simulink model "MARCH_demo"  (R2016a)
settings: Solver=FixedStepDiscrete  StartTime=0.0  StopTime=inf  FixedStep=0.001  RelTol=1e-3
InitFcn:
  | % Change dir to model location
  | cd(fileparts(which(bdroot)));
  | 
  | init_model
  | initialize_model_testingBlocks
StartFcn:
  | cd(fileparts(which(bdroot)));
StopFcn:
  | cd(fileparts(which(bdroot)));
model workspace (MAT data in the model file):
  localValue = 1
  targetValue = 0
undefined symbols (not defined in the file or in its folder): Hip_HAA, Left_Leg, Right_Leg
libraries: xpcethercatlib x54, slrtlib x7, aerolibanimutils x1, dspnetwork x1
CloseFcn:
  | cd(fileparts(which(bdroot)));
settings Model: Creator=march  LastModifiedBy=Nathan
settings SolverCC: EnableConcurrentExecution=on
settings DataIOCC: SaveFormat=StructureWithTime
settings OptimizationCC: BlockReduction=off  OptimizeBlockIOStorage=off  BufferReuse=off  GlobalBufferReuse=off  ExpressionFolding=off  LocalBlockOutputs=off
settings HardwareCC: ProdBitPerPointer=32  ProdLargestAtomicFloat=None  ProdWordSize=32  ProdLongLongMode=on  ProdHWDeviceType=Generic->32-bit x86 compatible
settings RTWCC: SystemTargetFile=slrt.tlc  TemplateMakefile=slrt_default_tmf  Description=Simulink Real-Time
settings SimulinkRealTimeCC: xPCisDownloadable=off  xPCisModelTimeout=off  xPCModelTimeoutSecs=30

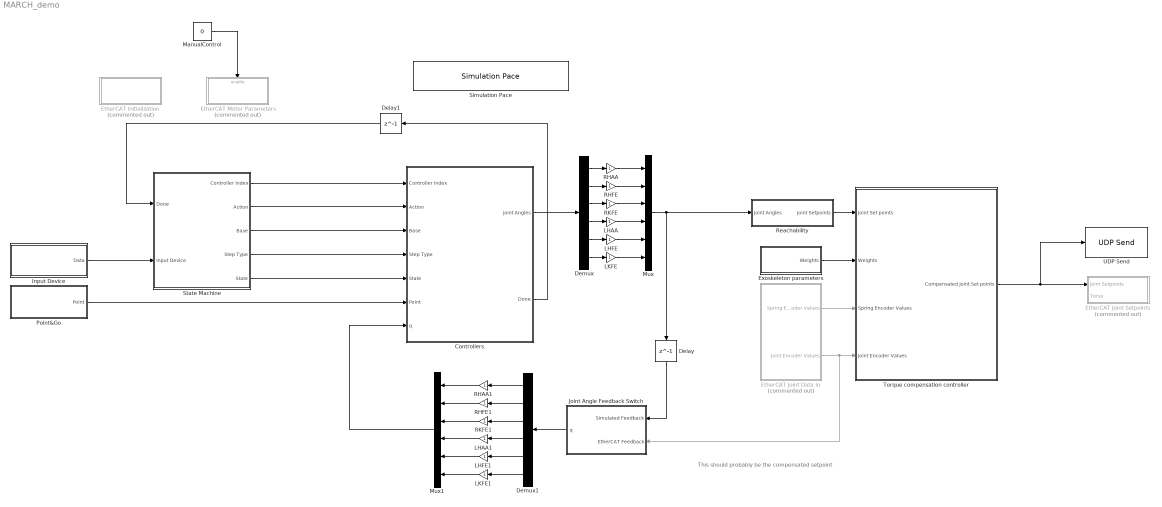
== system MARCH_demo ==
  note: This should probably be the compensated setpoint
  Controllers : Subsystem
  Delay : Delay  DelayLength=1
  Delay1 : Delay  DelayLength=1
  Demux : Demux  Outputs=6
  Demux1 : Demux  Outputs=6
  EtherCAT Initialization : Subsystem  Commented=on
  EtherCAT Joint Data In : Subsystem  Commented=on
  EtherCAT Joint Setpoints : Subsystem  Commented=on
  EtherCAT Motor Parameters : Subsystem  Commented=on
  Exoskeleton parameters : Subsystem
  Input Device : Subsystem
  Joint Angle Feedback Switch : Subsystem
  LHAA : Gain
  LHAA1 : Gain
  LHFE : Gain
  LHFE1 : Gain
  LKFE : Gain
  LKFE1 : Gain
  ManualControl : Constant  Value=0
  Mux : Mux  Inputs=6
  Mux1 : Mux  Inputs=6
  Point&Go : Subsystem
  RHAA : Gain
  RHAA1 : Gain
  RHFE : Gain
  RHFE1 : Gain
  RKFE : Gain
  RKFE1 : Gain
  Reachability : Subsystem
  Simulation Pace : aerolibanimutils/Simulation Pace  SimulationPace=1  SleepMode=MATLAB Thread  OutputPaceError=off  SampleTime=-1
  State Machine : Subsystem
  Torque compensation controller : Subsystem
  UDP Send : dspnetwork/UDP Send  remoteURL='127.0.0.1'  remotePort=25000  localURL='0.0.0.0'  localPortSource=Automatically determine  localPort=-1  sampletime=-1  separateLengthPort=0
  wires:
  Torque compensation controller/1(Compensated Joint Set points) -> UDP Send/1, EtherCAT Joint Setpoints/1(Joint Setpoints)
  Reachability/1(Joint Setpoints) -> Torque compensation controller/1(Joint Set points)
  EtherCAT Joint Data In/1(Spring Encoder Values) -> Torque compensation controller/3(Spring Encoder Values)
  EtherCAT Joint Data In/2(Joint Encoder Values) -> Joint Angle Feedback Switch/2(EtherCAT Feedback), Torque compensation controller/4(Joint Encoder Values)
  Exoskeleton parameters/1(Weights) -> Torque compensation controller/2(Weights)
  Delay/1 -> Joint Angle Feedback Switch/1(Simulated Feedback)
  Point&Go/1(Point) -> Controllers/6(Point)
  Input Device/1(Data) -> State Machine/2(Input Device)
  Controllers/2(Done) -> Delay1/1
  State Machine/4(Step Type) -> Controllers/4(Step Type)
  State Machine/2(Action) -> Controllers/2(Action)
  State Machine/3(Base) -> Controllers/3(Base)
  State Machine/1(Controller Index) -> Controllers/1(Controller Index)
  State Machine/5(State) -> Controllers/5(State)
  Delay1/1 -> State Machine/1(Done)
  Demux/1 -> RHAA/1
  Demux/2 -> RHFE/1
  Demux/3 -> RKFE/1
  Demux/4 -> LHAA/1
  Demux/5 -> LHFE/1
  Demux/6 -> LKFE/1
  Controllers/1(joint Angles) -> Demux/1
  Mux/1 -> Reachability/1(Joint Angles), Delay/1
  RHAA/1 -> Mux/1
  RHFE/1 -> Mux/2
  RKFE/1 -> Mux/3
  LHAA/1 -> Mux/4
  LHFE/1 -> Mux/5
  LKFE/1 -> Mux/6
  Demux1/1 -> RHAA1/1
  Demux1/2 -> RHFE1/1
  Demux1/3 -> RKFE1/1
  Demux1/4 -> LHAA1/1
  Demux1/5 -> LHFE1/1
  Demux1/6 -> LKFE1/1
  RHFE1/1 -> Mux1/2
  RKFE1/1 -> Mux1/3
  LHAA1/1 -> Mux1/4
  LHFE1/1 -> Mux1/5
  LKFE1/1 -> Mux1/6
  RHAA1/1 -> Mux1/1
  Joint Angle Feedback Switch/1(q) -> Demux1/1
  Mux1/1 -> Controllers/7(q)
  ManualControl/1 -> EtherCAT Motor Parameters/Enable

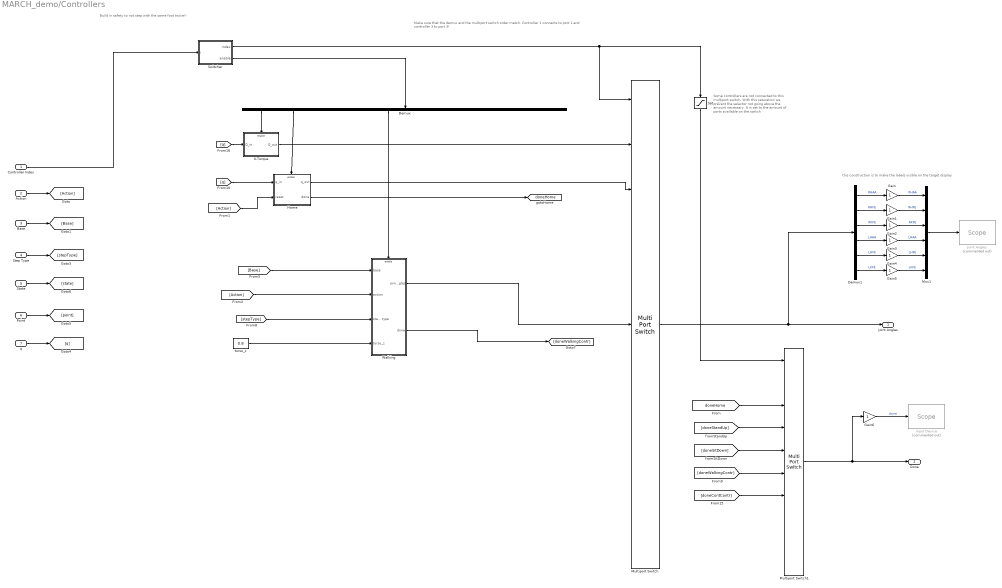
== system MARCH_demo/Controllers ==
  note: Some controllers are not connected to this multiport switch. With this saturation we prevent the selector not going above the amount necessary. It is set to the amount of ports available on the switch
  note: Build in safety to not step with the same
      | foot twice!!
  note: Make sure that the demux and the multiport switch order match.
      | Controller 1 connects to port 1 and controller 3 to port 3!
  note: this construction is to make the labels visible on the target display
  Controller Index : Inport
  Action : Inport  Port=2
  Base : Inport  Port=3
  Step Type : Inport  Port=4
  State : Inport  Port=5
  Point : Inport  Port=6
  q : Inport  Port=7
  0-Torque : Subsystem
  Demux : Demux  Outputs=10
  Demux1 : Demux  Outputs=6
  Gain{,1..6} (7 alike) : Gain
  Home : Subsystem
  Input Device : slrtlib/Displays and Logging/Scope   Commented=on  scopeno=4  scopetype=Target  autostart=on  viewmode=Graphical sliding  formatstr='%15.6f'  grid=on  ylimits=[0,0]  nosamples=25000  noprepostsamples=0  interleave=1  triggermode=FreeRun  triggersignal=1  trigsignalfromport=off  triggerlevel=0.0  triggerslope=Either  triggerscope=1  triggersample=0  filename=data.dat  mode=Lazy  writesize=512  autorestart=off  dynamicfilemode=off  maxwritefilesize=512*1024^2
  Joint Angles : slrtlib/Displays and Logging/Scope   Commented=on  scopeno=3  scopetype=Target  autostart=on  viewmode=Graphical sliding  formatstr='%15.6f'  grid=on  ylimits=[0,0]  nosamples=25000  noprepostsamples=0  interleave=1  triggermode=FreeRun  triggersignal=1  trigsignalfromport=off  triggerlevel=0.0  triggerslope=Either  triggerscope=1  triggersample=0  filename=data.dat  mode=Lazy  writesize=512  autorestart=off  dynamicfilemode=off  maxwritefilesize=512*1024^2
  Multiport Switch : MultiPortSwitch  Inputs=10
  Multiport Switch1 : MultiPortSwitch  Inputs=8  DataPortForDefault=Additional data port
  Mux1 : Mux  Inputs=6
  Saturation : Saturate  UpperLimit=8  LowerLimit=1
  Switcher : MATLAB Function  TreatAsAtomicUnit=on
  Walking : Subsystem
  torso_z : Constant  Value=0.8
  joint Angles : Outport
  Done : Outport  Port=2
  tag scope: doneHome=global
  wires:
  Switcher/1(index) -> Saturation/1, Multiport Switch/1
  Switcher/2(enable) -> Demux/1
  Multiport Switch1/1 -> Gain6/1, Done/1
  Saturation/1 -> Multiport Switch1/1
  Demux/1 -> 0-Torque/Enable
  Demux/5 -> Walking/Enable
  0-Torque/1(Q_out) -> Multiport Switch/2
  Home/1(q_out) -> Multiport Switch/3
  Walking/1(joint Angles) -> Multiport Switch/6
  Action/1 -> [Action]
  Base/1 -> [Base]
  Point/1 -> [point]
  q/1 -> [q]
  Step Type/1 -> [stepType]
  [Action] -> Walking/2(action)
  [Base] -> Walking/1(base)
  [stepType] -> Walking/3(step type)
  Walking/2(done) -> [doneWalkingContr]
  [doneWalkingContr] -> Multiport Switch1/6
  [doneContContr] -> Multiport Switch1/7
  State/1 -> [state]
  Home/2(done) -> [doneHome]
  [doneStandUp] -> Multiport Switch1/4
  Multiport Switch/1 -> joint Angles/1, Demux1/1
  Demux1/1 -> Gain/1  "RHAA"
  Demux1/2 -> Gain1/1  "RHFE"
  Demux1/3 -> Gain2/1  "RKFE"
  Demux1/4 -> Gain3/1  "LHAA"
  Demux1/5 -> Gain4/1  "LHFE"
  Demux1/6 -> Gain5/1  "LKFE"
  Mux1/1 -> Joint Angles/1
  Gain/1 -> Mux1/1  "RHAA"
  Gain1/1 -> Mux1/2  "RHFE"
  Gain2/1 -> Mux1/3  "RKFE"
  Gain3/1 -> Mux1/4  "LHAA"
  Gain4/1 -> Mux1/5  "LHFE"
  Gain5/1 -> Mux1/6  "LKFE"
  Gain6/1 -> Input Device/1  "done"
  [doneSitDown] -> Multiport Switch1/5
  Controller Index/1 -> Switcher/1(i)
  torso_z/1 -> Walking/4(torso_z)
  [q] -> 0-Torque/1(Q_in)
  [doneHome] -> Multiport Switch1/3
  [Action] -> Home/2(reset)
  [q] -> Home/1(q_in)
  Demux/2 -> Home/Enable

== system MARCH_demo/EtherCAT Initialization ==
  EtherCAT Init : xpcethercatlib/EtherCAT Init   Priority=0  config_file=C:\Users\march\Documents\Software\MATLAB\simulink-models\EtherCAT Config Files\full_setup_v1.0.xml  device_id=0  pci_bus=2  pci_slot=0  dctuning=0  enaDebug=off  enaDC=on  errLink=on  masterDbg=on  stateChgDbg=on  baseClock=off  masterCfg=off  logFile='c:\dbglog.txt'  sample_time=0.001000
  EtherCAT Init1 : xpcethercatlib/EtherCAT Init   Priority=0  config_file=C:\Users\march\Documents\Software\MATLAB\simulink-models\EtherCAT Config files\input_device.xml  device_id=1  pci_bus=3  pci_slot=0  dctuning=1  enaDebug=off  enaDC=on  errLink=on  masterDbg=on  stateChgDbg=on  baseClock=off  masterCfg=off  logFile='c:\dbglog.txt'  sample_time=0.001000
  Terminator : Terminator
  Terminator1 : Terminator
  wires:
  EtherCAT Init/1 -> Terminator/1
  EtherCAT Init1/1 -> Terminator1/1

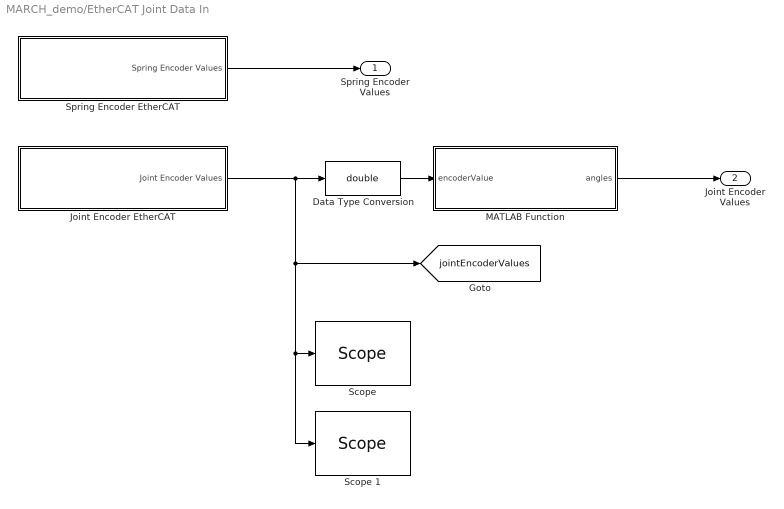
== system MARCH_demo/EtherCAT Joint Data In ==
  Data Type Conversion : DataTypeConversion  OutDataTypeStr=double
  Joint Encoder EtherCAT : Subsystem
  MATLAB Function : MATLAB Function  TreatAsAtomicUnit=on
  "Scope " : slrtlib/Displays and Logging/Scope   scopeno=6  scopetype=Target  autostart=on  viewmode=Graphical sliding  formatstr='%15.6f'  grid=on  ylimits=[0,0]  nosamples=25000  noprepostsamples=0  interleave=1  triggermode=FreeRun  triggersignal=1  trigsignalfromport=off  triggerlevel=0.0  triggerslope=Either  triggerscope=1  triggersample=0  filename=data.dat  mode=Lazy  writesize=512  autorestart=off  dynamicfilemode=off  maxwritefilesize=512*1024^2
  Scope 1 : slrtlib/Displays and Logging/Scope   scopeno=7  scopetype=Target  autostart=on  viewmode=Numerical  formatstr='%15.6f'  grid=on  ylimits=[0,0]  nosamples=3  noprepostsamples=0  interleave=1  triggermode=FreeRun  triggersignal=1  trigsignalfromport=off  triggerlevel=0.0  triggerslope=Either  triggerscope=1  triggersample=0  filename=data.dat  mode=Lazy  writesize=512  autorestart=off  dynamicfilemode=off  maxwritefilesize=512*1024^2
  Spring Encoder EtherCAT : Subsystem
  Spring Encoder Values : Outport
  Joint Encoder Values : Outport  Port=2
  tag scope: jointEncoderValues=global
  wires:
  Spring Encoder EtherCAT/1(Spring Encoder Values) -> Spring Encoder Values/1
  Joint Encoder EtherCAT/1(Joint Encoder Values) -> Data Type Conversion/1, Scope 1/1, "Scope "/1, [jointEncoderValues]
  MATLAB Function/1(angles) -> Joint Encoder Values/1
  Data Type Conversion/1 -> MATLAB Function/1(encoderValue)

== system MARCH_demo/EtherCAT Joint Setpoints ==
  Joint Setpoints : Inport
  Torso : Inport  Port=2
  Subsystem : Subsystem
  exoskeleton : Subsystem
  wires:
  Joint Setpoints/1 -> Subsystem/1(Joint Setpoints), exoskeleton/1(Joint setpoints)
  Torso/1 -> Subsystem/2(Torso)

== system MARCH_demo/EtherCAT Motor Parameters ==
  Enable : EnablePort
  Hips : Subsystem
  Left Leg : Subsystem
  Right Leg : Subsystem

== system MARCH_demo/Exoskeleton parameters ==
  Constant : Constant
  Weights : Outport
  wires:
  Constant/1 -> Weights/1

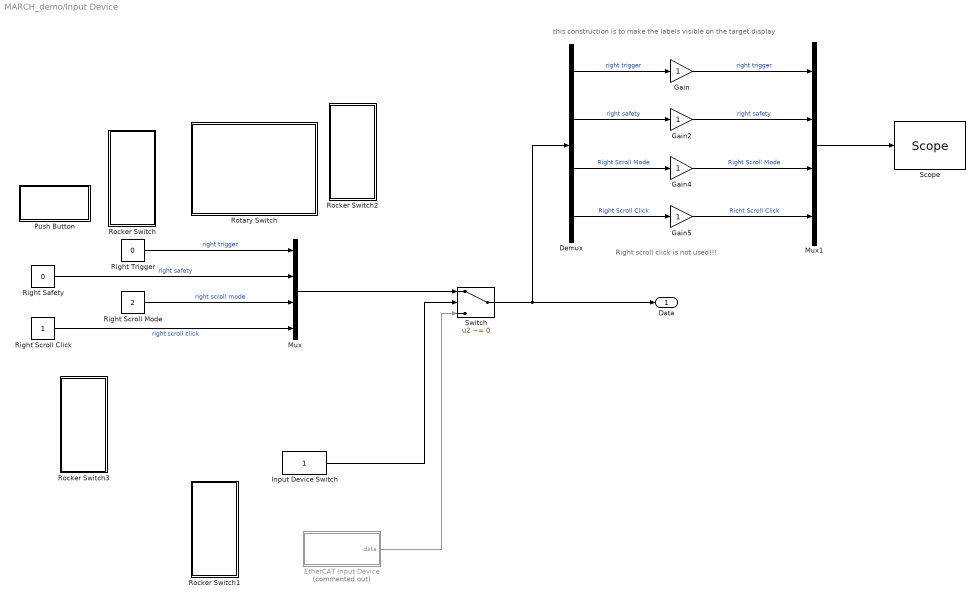
== system MARCH_demo/Input Device ==
  note: Right scroll click is not used!!!
  note: this construction is to make the labels visible on the target display
  Demux : Demux
  EtherCAT Input Device : Subsystem  Commented=on
  Gain{,2,4..5} (4 alike) : Gain
  Input Device Switch : Constant
  Mux : Mux
  Mux1 : Mux
  Push Button : Subsystem  DialogController=hmiCreateDDGDialog  IsWebBlock=on  mask(MWDashboardBlock){webBlockId=b5386708-d25b-47fc-ba10-cbba45de8cf4, webBlockType=pushbutton, ShowInLibBrwoser=on, ShowInitialText=on, HMISrcModelName=MARCH_demo}
      mask prompts: webBlockId "WebBlock Id"; webBlockType "WebBlock Type"; HMISrcModelName "Source Model"
      mask Help: helpview([docroot '/mapfiles/simulink.map'], 'hmi_push_button')
      mask Display:
      | model = bdroot(gcb);
      | if strcmp(get_param(model,'BlockDiagramType'), 'library')
      |     image([(matlabroot) '/toolbox/simulink/hmi/icons/PushButton.png']);
      | end
  Right Safety : Constant  Value=0
  Right Scroll Click : Constant
  Right Scroll Mode : Constant  Value=2
  Right Trigger : Constant  Value=0
  Rocker Switch : Subsystem  DialogController=hmiCreateDDGDialog  IsWebBlock=on  mask(MWDashboardBlock){webBlockId=45a61409-3ea3-4c23-95e6-fecf4e0aa3e0, webBlockType=rockerswitch, ShowInLibBrowser=on, ShowInitialText=on, HMISrcModelName=MARCH_demo}
      mask prompts: webBlockId "WebBlock Id"; webBlockType "WebBlock Type"; HMISrcModelName "Source Model"
      mask Help: helpview([docroot '/mapfiles/simulink.map'], 'hmi_rocker_switch')
      mask Display:
      | if strcmp(get_param(bdroot(gcb),'BlockDiagramType'), 'library')
      |     image([(matlabroot) '/toolbox/simulink/hmi/icons/RockerSwitch.png']);
      | end
  Rocker Switch1 : Subsystem  DialogController=hmiCreateDDGDialog  IsWebBlock=on  mask(MWDashboardBlock){webBlockId=cefc90cf-8074-4f09-bdc6-770b32cfa93a, webBlockType=rockerswitch, ShowInLibBrowser=on, ShowInitialText=on, HMISrcModelName=MARCH_demo}
      mask prompts: webBlockId "WebBlock Id"; webBlockType "WebBlock Type"; HMISrcModelName "Source Model"
      mask Help: helpview([docroot '/mapfiles/simulink.map'], 'hmi_rocker_switch')
      mask Display:
      | if strcmp(get_param(bdroot(gcb),'BlockDiagramType'), 'library')
      |     image([(matlabroot) '/toolbox/simulink/hmi/icons/RockerSwitch.png']);
      | end
  Rocker Switch2 : Subsystem  DialogController=hmiCreateDDGDialog  IsWebBlock=on  mask(MWDashboardBlock){webBlockId=9c410da0-0f2d-4180-a6e0-51db4255d255, webBlockType=rockerswitch, ShowInLibBrowser=on, ShowInitialText=on, HMISrcModelName=MARCH_demo}
      mask prompts: webBlockId "WebBlock Id"; webBlockType "WebBlock Type"; HMISrcModelName "Source Model"
      mask Help: helpview([docroot '/mapfiles/simulink.map'], 'hmi_rocker_switch')
      mask Display:
      | if strcmp(get_param(bdroot(gcb),'BlockDiagramType'), 'library')
      |     image([(matlabroot) '/toolbox/simulink/hmi/icons/RockerSwitch.png']);
      | end
  Rocker Switch3 : Subsystem  DialogController=hmiCreateDDGDialog  IsWebBlock=on  mask(MWDashboardBlock){webBlockId=f322042e-cbf0-407d-b585-24a2480925c8, webBlockType=rockerswitch, ShowInLibBrowser=on, ShowInitialText=on, HMISrcModelName=MARCH_demo}
      mask prompts: webBlockId "WebBlock Id"; webBlockType "WebBlock Type"; HMISrcModelName "Source Model"
      mask Help: helpview([docroot '/mapfiles/simulink.map'], 'hmi_rocker_switch')
      mask Display:
      | if strcmp(get_param(bdroot(gcb),'BlockDiagramType'), 'library')
      |     image([(matlabroot) '/toolbox/simulink/hmi/icons/RockerSwitch.png']);
      | end
  Rotary Switch : Subsystem  DialogController=hmiCreateDDGDialog  IsWebBlock=on  mask(MWDashboardBlock){webBlockId=2d14d417-f18b-4bf4-9f2c-b9e5fd3a8913, webBlockType=discreteknob, ShowInLibBrowser=on, ShowInitialText=on, HMISrcModelName=MARCH_demo}
      mask prompts: webBlockId "WebBlock Id"; webBlockType "WebBlock Type"; HMISrcModelName "Source Model"
      mask Help: helpview([docroot '/mapfiles/simulink.map'], 'hmi_rotary_switch')
      mask Display:
      | model = bdroot(gcb);
      | if strcmp(get_param(model,'BlockDiagramType'), 'library')
      |     image([(matlabroot) '/toolbox/simulink/hmi/icons/DiscreteKnob.png']);
      | end
  "Scope " : slrtlib/Displays and Logging/Scope   scopeno=1  scopetype=Target  autostart=on  viewmode=Numerical  formatstr='%15.6f'  grid=on  ylimits=[0,0]  nosamples=3  noprepostsamples=0  interleave=1  triggermode=FreeRun  triggersignal=1  trigsignalfromport=off  triggerlevel=0.0  triggerslope=Either  triggerscope=1  triggersample=0  filename=data.dat  mode=Lazy  writesize=512  autorestart=off  dynamicfilemode=off  maxwritefilesize=512*1024^2
  Switch : Switch  Criteria=u2 ~= 0
  Data : Outport
  wires:
  Input Device Switch/1 -> Switch/2
  EtherCAT Input Device/1(data) -> Switch/3
  Right Scroll Mode/1 -> Mux/3  "right scroll mode"
  Right Scroll Click/1 -> Mux/4  "right scroll click"
  Right Trigger/1 -> Mux/1  "right trigger"
  Right Safety/1 -> Mux/2  "right safety"
  Demux/1 -> Gain/1  "right trigger"
  Demux/2 -> Gain2/1  "right safety"
  Demux/3 -> Gain4/1  "Right Scroll Mode"
  Demux/4 -> Gain5/1  "Right Scroll Click"
  Gain/1 -> Mux1/1  "right trigger"
  Gain2/1 -> Mux1/2  "right safety"
  Gain4/1 -> Mux1/3  "Right Scroll Mode"
  Gain5/1 -> Mux1/4  "Richt Scroll Click"
  Switch/1 -> Data/1, Demux/1
  Mux/1 -> Switch/1
  Mux1/1 -> "Scope "/1

== system MARCH_demo/Joint Angle Feedback Switch ==
  Simulated Feedback : Inport
  EtherCAT Feedback : Inport  Port=2
  Local : Constant  Value=localValue
  Switch : Switch  Criteria=u2 ~= 0
  q : Outport
  wires:
  EtherCAT Feedback/1 -> Switch/3
  Switch/1 -> q/1
  Simulated Feedback/1 -> Switch/1
  Local/1 -> Switch/2

== system MARCH_demo/Point&Go ==
  note: For now, always use dummy point and go data even during target runs
  EtherCAT Point&Go : Subsystem  Commented=on
  Local : Constant  Value=localValue
  Point & Go Point : Constant  Value=[0.1 -0.3 0]
  Switch : Switch  Criteria=u2 ~= 0
  Point : Outport
  wires:
  EtherCAT Point&Go/1(Point&Go Data) -> Switch/3
  Local/1 -> Switch/2
  Switch/1 -> Point/1
  Point & Go Point/1 -> Switch/1

== system MARCH_demo/Reachability ==
  Joint Angles : Inport
  Data Type Conversion : DataTypeConversion  OutDataTypeStr=uint32
  MATLAB Function : MATLAB Function  Commented=on  TreatAsAtomicUnit=on
  Terminator2 : Terminator  Commented=on
  Joint Setpoints : Outport
  tag scope: jointSetpoints=global
  wires:
  MATLAB Function/2(err) -> Terminator2/1
  Data Type Conversion/1 -> [jointSetpoints]
  Joint Angles/1 -> Data Type Conversion/1, Joint Setpoints/1

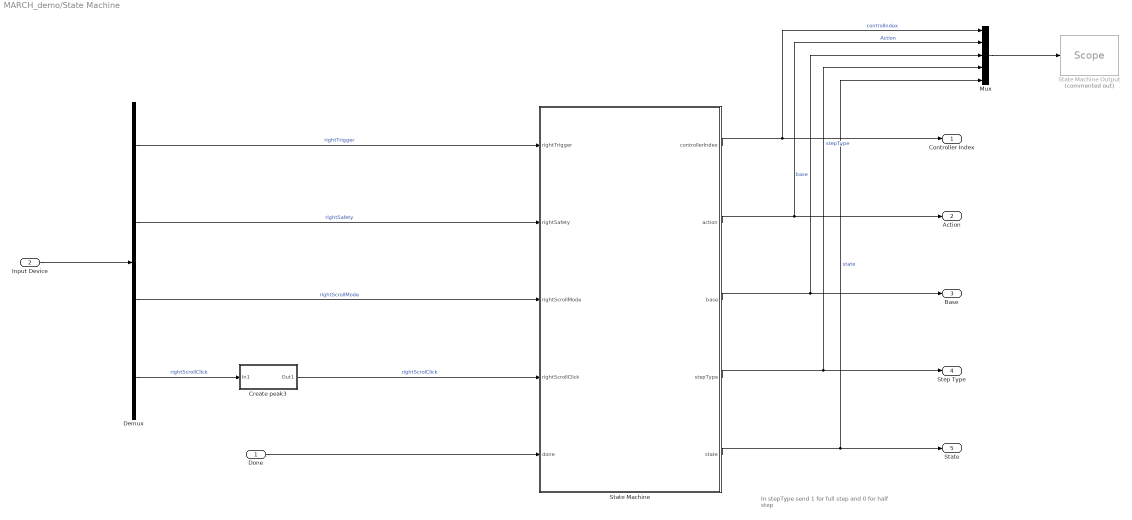
== system MARCH_demo/State Machine ==
  note: In stepType send 1 for full step and 0 for half step
  Done : Inport
  Input Device : Inport  Port=2
  Create peak3 : Subsystem
  Demux : Demux
  Mux : Mux  Inputs=5
  State Machine : Stateflow chart  TreatAsAtomicUnit=on
  State Machine Output : slrtlib/Displays and Logging/Scope   Commented=on  scopeno=2  scopetype=Target  autostart=on  viewmode=Numerical  formatstr='%15.6f'  grid=on  ylimits=[0,0]  nosamples=25  noprepostsamples=0  interleave=1  triggermode=FreeRun  triggersignal=1  trigsignalfromport=off  triggerlevel=0.0  triggerslope=Either  triggerscope=1  triggersample=0  filename=data.dat  mode=Lazy  writesize=512  autorestart=off  dynamicfilemode=off  maxwritefilesize=512*1024^2
  Controller Index : Outport
  Action : Outport  Port=2
  Base : Outport  Port=3
  Step Type : Outport  Port=4
  State : Outport  Port=5
  wires:
  Demux/2 -> State Machine/2(rightSafety)  "rightSafety"
  Demux/4 -> Create peak3/1(In1)  "rightScrollClick"
  Demux/1 -> State Machine/1(rightTrigger)  "rightTrigger"
  Create peak3/1(Out1) -> State Machine/4(rightScrollClick)  "rightScrolClick"
  Input Device/1 -> Demux/1
  Done/1 -> State Machine/5(done)
  State Machine/5(state) -> Mux/5, State/1  "state"
  State Machine/1(controllerIndex) -> Mux/1, Controller Index/1  "controlIndex"
  State Machine/2(action) -> Mux/2, Action/1  "Action"
  State Machine/3(base) -> Mux/3, Base/1  "base"
  State Machine/4(stepType) -> Mux/4, Step Type/1  "stepType"
  Mux/1 -> State Machine Output/1
  Demux/3 -> State Machine/3(rightScrollMode)  "rightScrollMode"

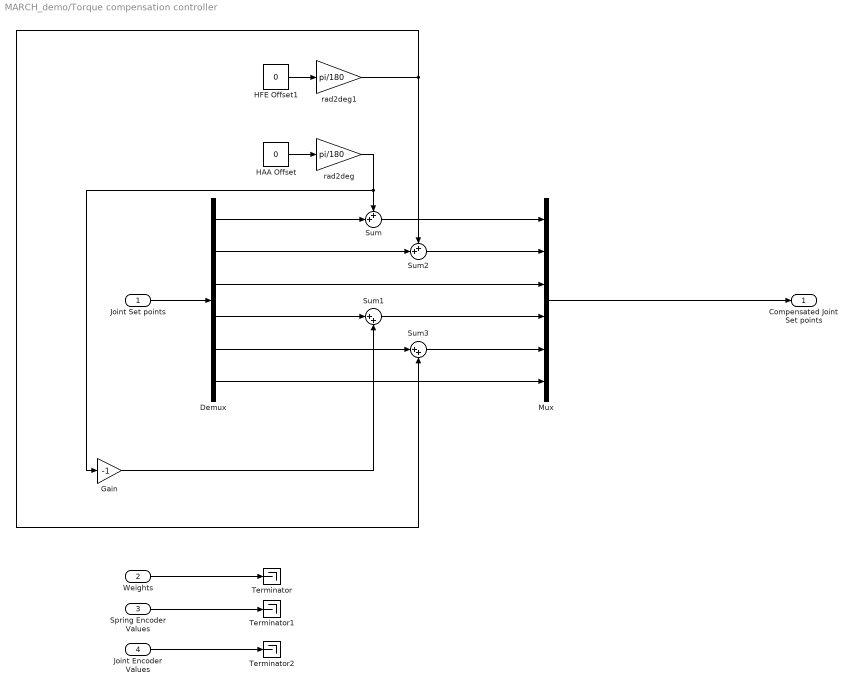
== system MARCH_demo/Torque compensation controller ==
  Joint Set points : Inport
  Weights : Inport  Port=2
  Spring Encoder Values : Inport  Port=3
  Joint Encoder Values : Inport  Port=4
  Demux : Demux  Outputs=6
  Gain : Gain  Gain=-1
  HAA Offset : Constant  Value=0
  HFE Offset1 : Constant  Value=0
  Mux : Mux  Inputs=6
  Sum : Sum  Inputs=++|
  Sum1 : Sum  Inputs=|++
  Sum2 : Sum  Inputs=++|
  Sum3 : Sum  Inputs=|++
  Terminator : Terminator
  Terminator1 : Terminator
  Terminator2 : Terminator
  rad2deg : Gain  Gain=pi/180
  rad2deg1 : Gain  Gain=pi/180
  Compensated Joint Set points : Outport
  wires:
  Joint Encoder Values/1 -> Terminator2/1
  Spring Encoder Values/1 -> Terminator1/1
  Weights/1 -> Terminator/1
  Joint Set points/1 -> Demux/1
  Demux/1 -> Sum/2
  Mux/1 -> Compensated Joint Set points/1
  Sum/1 -> Mux/1
  rad2deg/1 -> Gain/1, Sum/1
  HAA Offset/1 -> rad2deg/1
  Demux/2 -> Sum2/2
  Demux/3 -> Mux/3
  Sum1/1 -> Mux/4
  Demux/5 -> Sum3/1
  Demux/6 -> Mux/6
  Demux/4 -> Sum1/1
  Gain/1 -> Sum1/2
  HFE Offset1/1 -> rad2deg1/1
  Sum2/1 -> Mux/2
  Sum3/1 -> Mux/5
  rad2deg1/1 -> Sum2/1, Sum3/2

== system MARCH_demo/Controllers/0-Torque ==
  note: Since we don't control joint angles but motor velocity we just send dummy joint angles instead. This is a 1x6 vector of zeros.
  Q_in : Inport
  Enable : EnablePort  StatesWhenEnabling=reset
  Constant1 : Constant  Value=[0 0 0 0 0 0 ]  OutDataTypeStr=uint8
  Motor enable : Subsystem  Commented=on
  Q_out : Outport  InitialOutput=[0 0 0 0 0 0]
  wires:
  Q_in/1 -> Q_out/1
  Constant1/1 -> Motor enable/1(MotorEnableFlag)

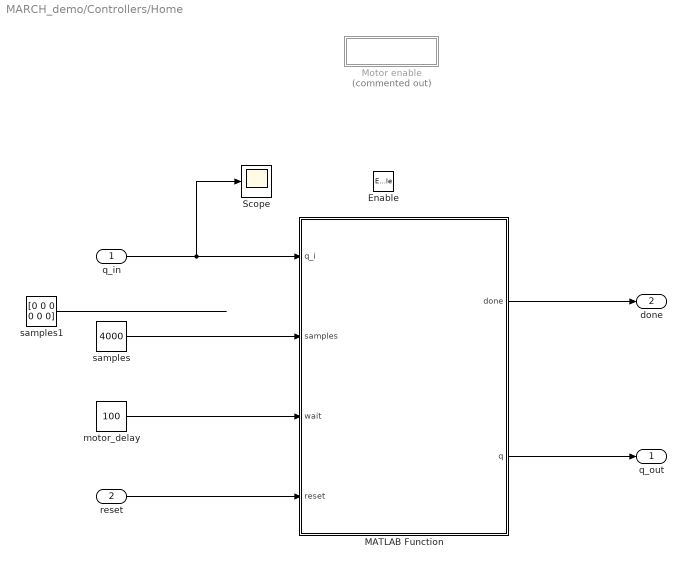
== system MARCH_demo/Controllers/Home ==
  q_in : Inport
  reset : Inport  Port=2
  Enable : EnablePort
  MATLAB Function : MATLAB Function  TreatAsAtomicUnit=on
  Motor enable : Subsystem  Commented=on
  Scope : Scope
  motor_delay : Constant  Value=100
  samples : Constant  Value=4000
  samples1 : Constant  Value=[0 0 0 0 0 0]
  q_out : Outport
  done : Outport  Port=2
  wires:
  MATLAB Function/1(done) -> done/1
  samples/1 -> MATLAB Function/2(samples)
  samples1/1 -> ?
  motor_delay/1 -> MATLAB Function/3(wait)
  MATLAB Function/2(q) -> q_out/1
  q_in/1 -> Scope/1, MATLAB Function/1(q_i)
  reset/1 -> MATLAB Function/4(reset)

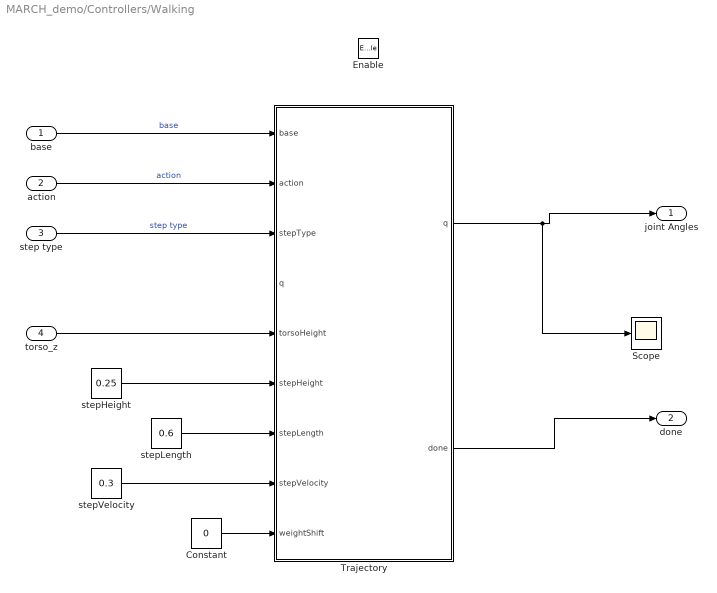
== system MARCH_demo/Controllers/Walking ==
  base : Inport
  action : Inport  Port=2
  step type : Inport  Port=3
  torso_z : Inport  Port=4
  Enable : EnablePort  StatesWhenEnabling=reset
  Constant : Constant  Value=0
  Scope : Scope
  Trajectory : MATLAB Function  TreatAsAtomicUnit=on
  stepHeight : Constant  Value=0.25
  stepLength : Constant  Value=0.6
  stepVelocity : Constant  Value=0.3
  joint Angles : Outport
  done : Outport  Port=2
  wires:
  Trajectory/1(q) -> Scope/1, joint Angles/1
  action/1 -> Trajectory/2(action)  "action"
  base/1 -> Trajectory/1(base)  "base"
  Trajectory/2(done) -> done/1
  step type/1 -> Trajectory/3(stepType)  "step type"
  stepHeight/1 -> Trajectory/6(stepHeight)
  stepLength/1 -> Trajectory/7(stepLength)
  stepVelocity/1 -> Trajectory/8(stepVelocity)
  Constant/1 -> Trajectory/9(weightShift)
  torso_z/1 -> Trajectory/5(torsoHeight)

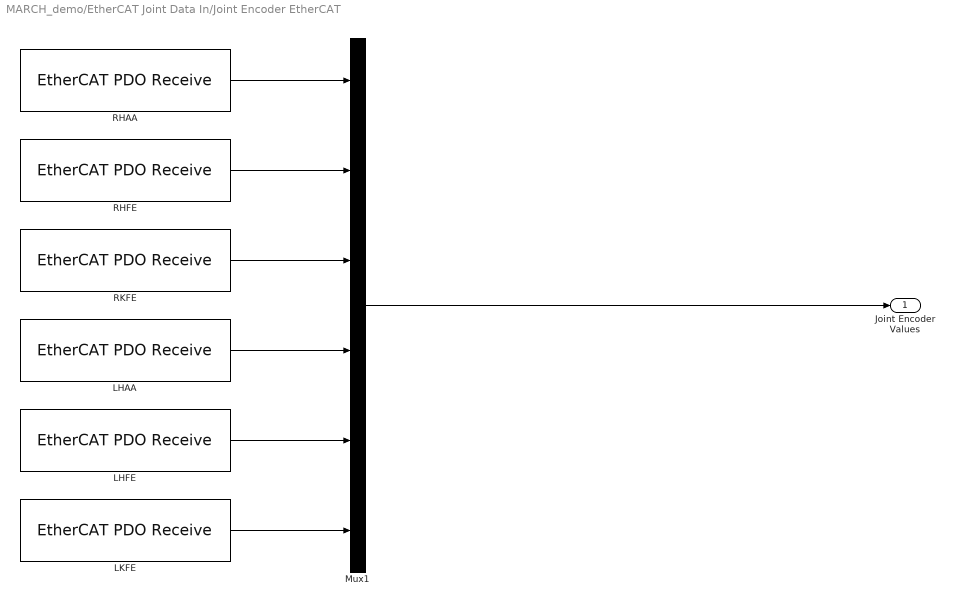
== system MARCH_demo/EtherCAT Joint Data In/Joint Encoder EtherCAT ==
  LHAA : xpcethercatlib/EtherCAT PDO Receive  Priority=2  sig_name=Hip_HAA.Inputs.L_jointAngle  sig_offset=208  sig_type=uint32  type_size=32  sig_dim=1  device_id=0  sample_time=0.001000
  LHFE : xpcethercatlib/EtherCAT PDO Receive  Priority=2  sig_name=Left_Leg.Inputs.H_springAngle  sig_offset=1176  sig_type=uint32  type_size=32  sig_dim=1  device_id=0  sample_time=0.001000
  LKFE : xpcethercatlib/EtherCAT PDO Receive  Priority=2  sig_name=Left_Leg.Inputs.K_jointAngle  sig_offset=1312  sig_type=uint32  type_size=32  sig_dim=1  device_id=0  sample_time=0.001000
  Mux1 : Mux  Inputs=6
  RHAA : xpcethercatlib/EtherCAT PDO Receive  Priority=2  sig_name=Hip_HAA.Inputs.R_jointAngle  sig_offset=688  sig_type=uint32  type_size=32  sig_dim=1  device_id=0  sample_time=0.001000
  RHFE : xpcethercatlib/EtherCAT PDO Receive  Priority=2  sig_name=Right_Leg.Inputs.H_jointAngle  sig_offset=1832  sig_type=uint32  type_size=32  sig_dim=1  device_id=0  sample_time=0.001000
  RKFE : xpcethercatlib/EtherCAT PDO Receive  Priority=2  sig_name=Right_Leg.Inputs.K_jointAngle  sig_offset=2000  sig_type=uint32  type_size=32  sig_dim=1  device_id=0  sample_time=0.001000
  Joint Encoder Values : Outport
  wires:
  RKFE/1 -> Mux1/3
  LHAA/1 -> Mux1/4
  RHFE/1 -> Mux1/2
  RHAA/1 -> Mux1/1
  LHFE/1 -> Mux1/5
  LKFE/1 -> Mux1/6
  Mux1/1 -> Joint Encoder Values/1

== system MARCH_demo/EtherCAT Joint Data In/Spring Encoder EtherCAT ==
  LHAA : xpcethercatlib/EtherCAT PDO Receive  Priority=2  sig_name=Hip_HAA.Inputs.L_springAngle  sig_offset=240  sig_type=uint32  type_size=32  sig_dim=1  device_id=0  sample_time=0.001000
  LHFE : xpcethercatlib/EtherCAT PDO Receive  Priority=2  sig_name=Left_Leg.Inputs.H_springAngle  sig_offset=1176  sig_type=uint32  type_size=32  sig_dim=1  device_id=0  sample_time=0.001000
  LKFE : xpcethercatlib/EtherCAT PDO Receive  Priority=2  sig_name=Left_Leg.Inputs.K_springAngle  sig_offset=1344  sig_type=uint32  type_size=32  sig_dim=1  device_id=0  sample_time=0.001000
  Mux : Mux  Inputs=6
  RHAA : xpcethercatlib/EtherCAT PDO Receive  Priority=2  sig_name=Hip_HAA.Inputs.R_springAngle  sig_offset=720  sig_type=uint32  type_size=32  sig_dim=1  device_id=0  sample_time=0.001000
  RHFE : xpcethercatlib/EtherCAT PDO Receive  Priority=2  sig_name=Right_Leg.Inputs.H_springAngle  sig_offset=1864  sig_type=uint32  type_size=32  sig_dim=1  device_id=0  sample_time=0.001000
  RKFE : xpcethercatlib/EtherCAT PDO Receive  Priority=2  sig_name=Right_Leg.Inputs.K_springAngle  sig_offset=2032  sig_type=uint32  type_size=32  sig_dim=1  device_id=0  sample_time=0.001000
  Spring Encoder Values : Outport
  wires:
  RKFE/1 -> Mux/3
  LHFE/1 -> Mux/5
  Mux/1 -> Spring Encoder Values/1
  LKFE/1 -> Mux/6
  RHFE/1 -> Mux/2
  RHAA/1 -> Mux/1
  LHAA/1 -> Mux/4

== system MARCH_demo/EtherCAT Joint Setpoints/Subsystem ==
  Joint Setpoints : Inport
  Torso : Inport  Port=2
  Data Type Conversion : DataTypeConversion  OutDataTypeStr=uint32
  Data Type Conversion1 : DataTypeConversion  OutDataTypeStr=uint32
  tag scope: correctedJointSetpoints=global, torso=global
  wires:
  Joint Setpoints/1 -> Data Type Conversion/1
  Torso/1 -> Data Type Conversion1/1
  Data Type Conversion/1 -> [correctedJointSetpoints]
  Data Type Conversion1/1 -> [torso]

== system MARCH_demo/EtherCAT Joint Setpoints/exoskeleton ==
  Joint setpoints : Inport
  Data Type Conversion : DataTypeConversion  OutDataTypeStr=uint32
  EtherCAT Joint Communication : Subsystem
  MATLAB Function : MATLAB Function  TreatAsAtomicUnit=on
  "Scope " : slrtlib/Displays and Logging/Scope   scopeno=5  scopetype=Target  autostart=on  viewmode=Graphical sliding  formatstr='%15.6f'  grid=on  ylimits=[0,0]  nosamples=25000  noprepostsamples=0  interleave=1  triggermode=FreeRun  triggersignal=1  trigsignalfromport=off  triggerlevel=0.0  triggerslope=Either  triggerscope=1  triggersample=0  filename=data.dat  mode=Lazy  writesize=512  autorestart=off  dynamicfilemode=off  maxwritefilesize=512*1024^2
  wires:
  Data Type Conversion/1 -> EtherCAT Joint Communication/1(Joint Setpoints)
  Joint setpoints/1 -> MATLAB Function/1(jointAngle)
  MATLAB Function/1(encVal) -> "Scope "/1, Data Type Conversion/1

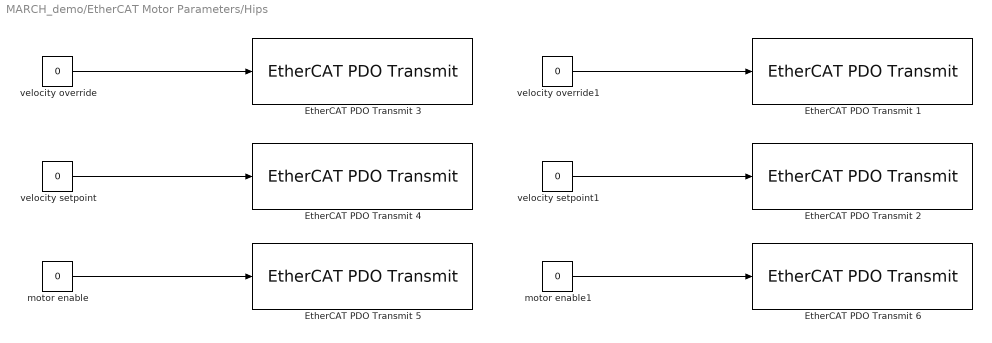
== system MARCH_demo/EtherCAT Motor Parameters/Hips ==
  EtherCAT PDO Transmit 1 : xpcethercatlib/EtherCAT PDO Transmit   Priority=3  sig_name=Hip_HAA.Outputs.R_data[4]  sig_offset=784  sig_type=int32  type_size=32  sig_dim=1  device_id=0  sample_time=0.001000
  EtherCAT PDO Transmit 2 : xpcethercatlib/EtherCAT PDO Transmit   Priority=3  sig_name=Hip_HAA.Outputs.R_velocitySetPoint  sig_offset=512  sig_type=int16  type_size=16  sig_dim=1  device_id=0  sample_time=0.001000
  EtherCAT PDO Transmit 3 : xpcethercatlib/EtherCAT PDO Transmit   Priority=3  sig_name=Hip_HAA.Outputs.L_data[4]  sig_offset=480  sig_type=int32  type_size=32  sig_dim=1  device_id=0  sample_time=0.001000
  EtherCAT PDO Transmit 4 : xpcethercatlib/EtherCAT PDO Transmit   Priority=3  sig_name=Hip_HAA.Outputs.L_velocitySetPoint  sig_offset=208  sig_type=int16  type_size=16  sig_dim=1  device_id=0  sample_time=0.001000
  EtherCAT PDO Transmit 5 : xpcethercatlib/EtherCAT PDO Transmit   Priority=3  sig_name=Hip_HAA.Outputs.L_motorEnable  sig_offset=256  sig_type=uint8  type_size=8  sig_dim=1  device_id=0  sample_time=0.001000
  EtherCAT PDO Transmit 6 : xpcethercatlib/EtherCAT PDO Transmit   Priority=3  sig_name=Hip_HAA.Outputs.R_motorEnable  sig_offset=560  sig_type=uint8  type_size=8  sig_dim=1  device_id=0  sample_time=0.001000
  motor enable : Constant  Value=0  OutDataTypeStr=uint8
  motor enable1 : Constant  Value=0  OutDataTypeStr=uint8
  velocity override : Constant  Value=0  OutDataTypeStr=int32
  velocity override1 : Constant  Value=0  OutDataTypeStr=int32
  velocity setpoint : Constant  Value=0  OutDataTypeStr=int16
  velocity setpoint1 : Constant  Value=0  OutDataTypeStr=int16
  wires:
  motor enable/1 -> EtherCAT PDO Transmit 5/1
  velocity override/1 -> EtherCAT PDO Transmit 3/1
  velocity setpoint/1 -> EtherCAT PDO Transmit 4/1
  motor enable1/1 -> EtherCAT PDO Transmit 6/1
  velocity override1/1 -> EtherCAT PDO Transmit 1/1
  velocity setpoint1/1 -> EtherCAT PDO Transmit 2/1

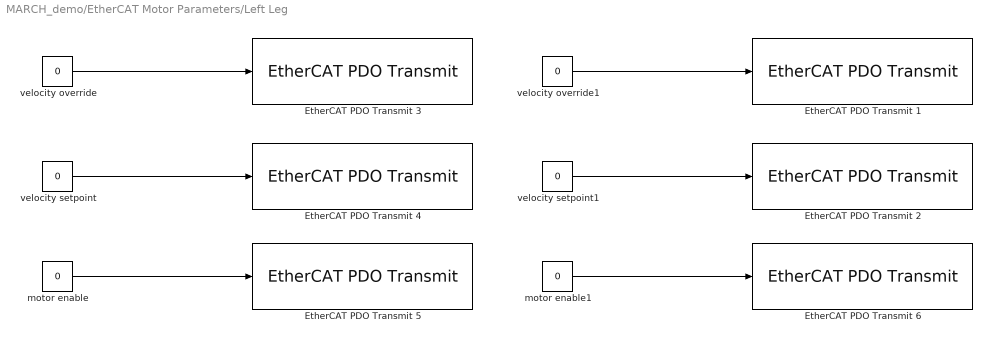
== system MARCH_demo/EtherCAT Motor Parameters/Left Leg ==
  EtherCAT PDO Transmit 1 : xpcethercatlib/EtherCAT PDO Transmit   Priority=3  sig_name=Left_Leg.Outputs.K_data[4]  sig_offset=1688  sig_type=int32  type_size=32  sig_dim=1  device_id=0  sample_time=0.001000
  EtherCAT PDO Transmit 2 : xpcethercatlib/EtherCAT PDO Transmit   Priority=3  sig_name=Left_Leg.Outputs.K_velocitySetPoint  sig_offset=1432  sig_type=int16  type_size=16  sig_dim=1  device_id=0  sample_time=0.001000
  EtherCAT PDO Transmit 3 : xpcethercatlib/EtherCAT PDO Transmit   Priority=3  sig_name=Left_Leg.Outputs.H_data[4]  sig_offset=1400  sig_type=int32  type_size=32  sig_dim=1  device_id=0  sample_time=0.001000
  EtherCAT PDO Transmit 4 : xpcethercatlib/EtherCAT PDO Transmit   Priority=3  sig_name=Left_Leg.Outputs.H_velocitySetPoint  sig_offset=1144  sig_type=int16  type_size=16  sig_dim=1  device_id=0  sample_time=0.001000
  EtherCAT PDO Transmit 5 : xpcethercatlib/EtherCAT PDO Transmit   Priority=3  sig_name=Left_Leg.Outputs.H_motorEnable  sig_offset=1192  sig_type=uint8  type_size=8  sig_dim=1  device_id=0  sample_time=0.001000
  EtherCAT PDO Transmit 6 : xpcethercatlib/EtherCAT PDO Transmit   Priority=3  sig_name=Left_Leg.Outputs.K_motorEnable  sig_offset=1480  sig_type=uint8  type_size=8  sig_dim=1  device_id=0  sample_time=0.001000
  motor enable : Constant  Value=0  OutDataTypeStr=uint8
  motor enable1 : Constant  Value=0  OutDataTypeStr=uint8
  velocity override : Constant  Value=0  OutDataTypeStr=int32
  velocity override1 : Constant  Value=0  OutDataTypeStr=int32
  velocity setpoint : Constant  Value=0  OutDataTypeStr=int16
  velocity setpoint1 : Constant  Value=0  OutDataTypeStr=int16
  wires:
  motor enable/1 -> EtherCAT PDO Transmit 5/1
  velocity override/1 -> EtherCAT PDO Transmit 3/1
  velocity setpoint/1 -> EtherCAT PDO Transmit 4/1
  motor enable1/1 -> EtherCAT PDO Transmit 6/1
  velocity override1/1 -> EtherCAT PDO Transmit 1/1
  velocity setpoint1/1 -> EtherCAT PDO Transmit 2/1

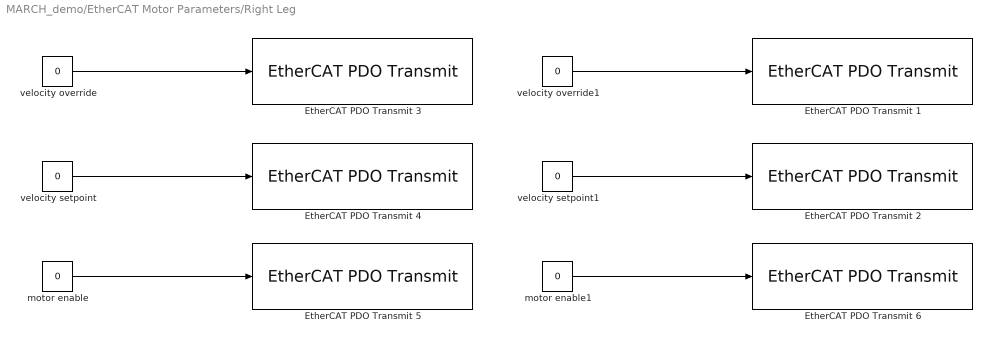
== system MARCH_demo/EtherCAT Motor Parameters/Right Leg ==
  EtherCAT PDO Transmit 1 : xpcethercatlib/EtherCAT PDO Transmit   Priority=3  sig_name=Right_Leg.Outputs.K_data[4]  sig_offset=2376  sig_type=int32  type_size=32  sig_dim=1  device_id=0  sample_time=0.001000
  EtherCAT PDO Transmit 2 : xpcethercatlib/EtherCAT PDO Transmit   Priority=3  sig_name=Right_Leg.Outputs.K_velocitySetPoint  sig_offset=2120  sig_type=int16  type_size=16  sig_dim=1  device_id=0  sample_time=0.001000
  EtherCAT PDO Transmit 3 : xpcethercatlib/EtherCAT PDO Transmit   Priority=3  sig_name=Right_Leg.Outputs.H_data[4]  sig_offset=2088  sig_type=int32  type_size=32  sig_dim=1  device_id=0  sample_time=0.001000
  EtherCAT PDO Transmit 4 : xpcethercatlib/EtherCAT PDO Transmit   Priority=3  sig_name=Right_Leg.Outputs.H_velocitySetPoint  sig_offset=1832  sig_type=int16  type_size=16  sig_dim=1  device_id=0  sample_time=0.001000
  EtherCAT PDO Transmit 5 : xpcethercatlib/EtherCAT PDO Transmit   Priority=3  sig_name=Right_Leg.Outputs.H_motorEnable  sig_offset=1880  sig_type=uint8  type_size=8  sig_dim=1  device_id=0  sample_time=0.001000
  EtherCAT PDO Transmit 6 : xpcethercatlib/EtherCAT PDO Transmit   Priority=3  sig_name=Right_Leg.Outputs.K_motorEnable  sig_offset=2168  sig_type=uint8  type_size=8  sig_dim=1  device_id=0  sample_time=0.001000
  motor enable : Constant  Value=0  OutDataTypeStr=uint8
  motor enable1 : Constant  Value=0  OutDataTypeStr=uint8
  velocity override : Constant  Value=0  OutDataTypeStr=int32
  velocity override1 : Constant  Value=0  OutDataTypeStr=int32
  velocity setpoint : Constant  Value=0  OutDataTypeStr=int16
  velocity setpoint1 : Constant  Value=0  OutDataTypeStr=int16
  wires:
  motor enable/1 -> EtherCAT PDO Transmit 5/1
  velocity override/1 -> EtherCAT PDO Transmit 3/1
  velocity setpoint/1 -> EtherCAT PDO Transmit 4/1
  motor enable1/1 -> EtherCAT PDO Transmit 6/1
  velocity override1/1 -> EtherCAT PDO Transmit 1/1
  velocity setpoint1/1 -> EtherCAT PDO Transmit 2/1

== system MARCH_demo/Input Device/EtherCAT Input Device ==
  note: Dummy scroll click because old legacy code. This doesn't do anything!
  Constant : Constant  Value=0  OutDataTypeStr=uint8
  EtherCAT Safety : xpcethercatlib/EtherCAT PDO Receive  Priority=2  sig_name=Box 1 (FB1111 SPI-Slave).Inputs.safety  sig_offset=208  sig_type=uint8  type_size=8  sig_dim=1  device_id=1  sample_time=0.001000
  EtherCAT State : xpcethercatlib/EtherCAT PDO Receive  Priority=2  sig_name=Box 1 (FB1111 SPI-Slave).Inputs.state  sig_offset=224  sig_type=uint8  type_size=8  sig_dim=1  device_id=1  sample_time=0.001000
  EtherCAT Trigger : xpcethercatlib/EtherCAT PDO Receive  Priority=2  sig_name=Box 1 (FB1111 SPI-Slave).Inputs.trigger  sig_offset=216  sig_type=uint8  type_size=8  sig_dim=1  device_id=1  sample_time=0.001000
  Mux : Mux
  data : Outport
  wires:
  EtherCAT Safety/1 -> Mux/2  "safety"
  EtherCAT State/1 -> Mux/3  "state"
  EtherCAT Trigger/1 -> Mux/1  "trigger"
  Constant/1 -> Mux/4
  Mux/1 -> data/1

== system MARCH_demo/Input Device/Push Button ==

== system MARCH_demo/Input Device/Rocker Switch ==

== system MARCH_demo/Input Device/Rocker Switch1 ==

== system MARCH_demo/Input Device/Rocker Switch2 ==

== system MARCH_demo/Input Device/Rocker Switch3 ==

== system MARCH_demo/Input Device/Rotary Switch ==

== system MARCH_demo/Point&Go/EtherCAT Point&Go ==
  EtherCAT PDO Receive : xpcethercatlib/EtherCAT PDO Receive  Priority=2  sig_name=Hip_HAA.Inputs.R_crutchProximity[0]  sig_offset=984  sig_type=uint32  type_size=32  sig_dim=1  device_id=0  sample_time=0.001000
  Point&Go Data : Outport
  wires:
  EtherCAT PDO Receive/1 -> Point&Go Data/1

== system MARCH_demo/State Machine/Create peak3 ==
  In1 : Inport
  Delay : Delay  DelayLength=1
  Greater than 0 : MATLAB Function  TreatAsAtomicUnit=on
  Sum : Sum  Inputs=|-+
  Out1 : Outport
  wires:
  Sum/1 -> Greater than 0/1(peak)
  In1/1 -> Sum/2, Delay/1
  Delay/1 -> Sum/1
  Greater than 0/1(signal) -> Out1/1

== system MARCH_demo/Controllers/0-Torque/Motor enable ==
  MotorEnableFlag : Inport
  Demux : Demux  Outputs=6
  Enable LHAA : xpcethercatlib/EtherCAT PDO Transmit   Priority=3  sig_name=Hip_HAA.Outputs.L_motorEnable  sig_offset=256  sig_type=uint8  type_size=8  sig_dim=1  device_id=0  sample_time=0.001000
  Enable LHFE : xpcethercatlib/EtherCAT PDO Transmit   Priority=3  sig_name=Left_Leg.Outputs.H_motorEnable  sig_offset=1192  sig_type=uint8  type_size=8  sig_dim=1  device_id=0  sample_time=0.001000
  Enable LKFE : xpcethercatlib/EtherCAT PDO Transmit   Priority=3  sig_name=Left_Leg.Outputs.K_motorEnable  sig_offset=1480  sig_type=uint8  type_size=8  sig_dim=1  device_id=0  sample_time=0.001000
  Enable RHAA : xpcethercatlib/EtherCAT PDO Transmit   Priority=3  sig_name=Hip_HAA.Outputs.R_motorEnable  sig_offset=560  sig_type=uint8  type_size=8  sig_dim=1  device_id=0  sample_time=0.001000
  Enable RHFE : xpcethercatlib/EtherCAT PDO Transmit   Priority=3  sig_name=Right_Leg.Outputs.H_motorEnable  sig_offset=1880  sig_type=uint8  type_size=8  sig_dim=1  device_id=0  sample_time=0.001000
  Enable RKFE : xpcethercatlib/EtherCAT PDO Transmit   Priority=3  sig_name=Right_Leg.Outputs.K_motorEnable  sig_offset=2168  sig_type=uint8  type_size=8  sig_dim=1  device_id=0  sample_time=0.001000
  wires:
  Demux/3 -> Enable RKFE/1
  Demux/6 -> Enable LKFE/1
  Demux/5 -> Enable LHFE/1
  Demux/2 -> Enable RHFE/1
  MotorEnableFlag/1 -> Demux/1
  Demux/4 -> Enable LHAA/1
  Demux/1 -> Enable RHAA/1

== system MARCH_demo/Controllers/Home/Motor enable ==
  Demux : Demux  Outputs=6
  Enable LHAA : xpcethercatlib/EtherCAT PDO Transmit   Priority=3  sig_name=Hip_HAA.Outputs.L_motorEnable  sig_offset=256  sig_type=uint8  type_size=8  sig_dim=1  device_id=0  sample_time=0.001000
  Enable LHFE : xpcethercatlib/EtherCAT PDO Transmit   Priority=3  sig_name=Left_Leg.Outputs.H_motorEnable  sig_offset=1192  sig_type=uint8  type_size=8  sig_dim=1  device_id=0  sample_time=0.001000
  Enable LKFE : xpcethercatlib/EtherCAT PDO Transmit   Priority=3  sig_name=Left_Leg.Outputs.K_motorEnable  sig_offset=1480  sig_type=uint8  type_size=8  sig_dim=1  device_id=0  sample_time=0.001000
  Enable RHAA : xpcethercatlib/EtherCAT PDO Transmit   Priority=3  sig_name=Hip_HAA.Outputs.R_motorEnable  sig_offset=560  sig_type=uint8  type_size=8  sig_dim=1  device_id=0  sample_time=0.001000
  Enable RHFE : xpcethercatlib/EtherCAT PDO Transmit   Priority=3  sig_name=Right_Leg.Outputs.H_motorEnable  sig_offset=1880  sig_type=uint8  type_size=8  sig_dim=1  device_id=0  sample_time=0.001000
  Enable RKFE : xpcethercatlib/EtherCAT PDO Transmit   Priority=3  sig_name=Right_Leg.Outputs.K_motorEnable  sig_offset=2168  sig_type=uint8  type_size=8  sig_dim=1  device_id=0  sample_time=0.001000
  flag : Constant  Value=[1 1 1 1 1 1]  OutDataTypeStr=uint8
  wires:
  Demux/3 -> Enable RKFE/1
  Demux/6 -> Enable LKFE/1
  Demux/5 -> Enable LHFE/1
  Demux/2 -> Enable RHFE/1
  flag/1 -> Demux/1
  Demux/4 -> Enable LHAA/1
  Demux/1 -> Enable RHAA/1

== system MARCH_demo/EtherCAT Joint Setpoints/exoskeleton/EtherCAT Joint Communication ==
  Joint Setpoints : Inport
  Demux : Demux  Outputs=6
  "EtherCAT PDO Transmit " : xpcethercatlib/EtherCAT PDO Transmit   Priority=3  sig_name=Hip_HAA.Outputs.R_jointSetPoint  sig_offset=528  sig_type=uint32  type_size=32  sig_dim=1  device_id=0  sample_time=0.001000
  EtherCAT PDO Transmit 1 : xpcethercatlib/EtherCAT PDO Transmit   Priority=3  sig_name=Right_Leg.Outputs.H_jointSetPoint  sig_offset=1848  sig_type=uint32  type_size=32  sig_dim=1  device_id=0  sample_time=0.001000
  EtherCAT PDO Transmit 2 : xpcethercatlib/EtherCAT PDO Transmit   Priority=3  sig_name=Right_Leg.Outputs.K_jointSetPoint  sig_offset=2136  sig_type=uint32  type_size=32  sig_dim=1  device_id=0  sample_time=0.001000
  EtherCAT PDO Transmit 3 : xpcethercatlib/EtherCAT PDO Transmit   Priority=3  sig_name=Hip_HAA.Outputs.L_jointSetPoint  sig_offset=224  sig_type=uint32  type_size=32  sig_dim=1  device_id=0  sample_time=0.001000
  EtherCAT PDO Transmit 4 : xpcethercatlib/EtherCAT PDO Transmit   Priority=3  sig_name=Left_Leg.Outputs.H_jointSetPoint  sig_offset=1160  sig_type=uint32  type_size=32  sig_dim=1  device_id=0  sample_time=0.001000
  EtherCAT PDO Transmit 5 : xpcethercatlib/EtherCAT PDO Transmit   Priority=3  sig_name=Left_Leg.Outputs.K_jointSetPoint  sig_offset=1448  sig_type=uint32  type_size=32  sig_dim=1  device_id=0  sample_time=0.001000
  wires:
  Demux/5 -> EtherCAT PDO Transmit 4/1
  Demux/6 -> EtherCAT PDO Transmit 5/1
  Demux/4 -> EtherCAT PDO Transmit 3/1
  Demux/1 -> "EtherCAT PDO Transmit "/1
  Demux/2 -> EtherCAT PDO Transmit 1/1
  Joint Setpoints/1 -> Demux/1
  Demux/3 -> EtherCAT PDO Transmit 2/1

== matlab function MARCH_demo/Reachability/MATLAB Function ==
  data: q input size=6; q_out output size=6; err output size=6
function [q_out, err] = fcn(q)

joint_limit_min = [-20 -109 -3 -23 -109 -3]'/180*pi;
joint_limit_max = [23 21 121 20 21 121]'/180*pi;

n = size(q,2);
%% Check if all joints are within limits

err = imag(q)~=0 | q<repmat(joint_limit_min,n,1) | q>repmat(joint_limit_max,n,1);
q_out = q;

== matlab function MARCH_demo/Controllers/Switcher ==
  data: index output; i input; enable output
function [index, enable]= fcn(i)
%#codegen

% This function is supposed to take a state and switch between controllers.
% Currently it directly routes the input argument as the index. In the
% future this can be something different so I have left it open for
% future modifications.

% The u vector represents the controllers. When the vector consists out of
% zeros it will not enable any controller. In the case that an index is set
% to a non zero value, the controller which belongs to that index will be
% enabled.
u = zeros(10,1);

u(i) = 2;

index = i;
enable = u;

== matlab function MARCH_demo/EtherCAT Joint Data In/MATLAB Function ==
  data: encoderValue input; angles output; par parameter
function angles = convertToJointAngles(encoderValue, par)
angles = zeros(6,1);

for i = 1:6
    angles(i) = enc2rad(encoderValue(i), i, par);
end

== matlab function MARCH_demo/Controllers/Walking/Trajectory ==
  data: base input; q output; done output; action input; stepType input; q input size=[1 6]; torsoHeight input; stepHeight input; stepLength input; stepVelocity input; weightShift input
function [q,done]= fcn(base,action,stepType, q, torsoHeight,stepHeight, stepLength, stepVelocity, weightShift)
%#codegen

persistent r splineCtrl i triggerPersistent torsoTrajectory trajectory hold fullWeightShift timeCurve weightShiftRatio;

%% Initialize all variables
if(isempty(splineCtrl))
    splineCtrl = splineController();
end

if(isempty(fullWeightShift))
    fullWeightShift = 0;
end

if(isempty(stepType))
    stepType = 0;
end

if(isempty(r))
    % Get frequency of the model
    r = robotics();
    r.base = base;
    timeCurve = [0 0 0];
end

if(isempty(hold))
    hold = 0;
end

if(isempty(i))
    i = 0;
end

if(isempty(triggerPersistent))
    triggerPersistent = action;
end


if(isempty(trajectory))
    trajectory = [0 0 0];
    torsoTrajectory = [0 0 0];
end

if(isempty(weightShiftRatio))
    weightShiftRatio = 0;
end
    
%% Logic
% Only run this for the beginning of the swing
done = 0;

% Reset values if trigger is toggled.
if(triggerPersistent ~= action)
    r.base = base;
    i = 0;
    hold = 0;
    triggerPersistent = action;
end

% Hold exoskeleton in same position after a single step
if(hold)
    q = r.q;
    done = 1;
    return
end

if(~i)
    % Foot Trajectory
    splineCtrl.method('circle');
    splineCtrl.setStepHeight(stepHeight).setStepLength(stepLength);
    if(~stepType)
        trajectory = splineCtrl.method('circle').setVelocity(stepVelocity).getHalfStep();
    else
        trajectory = splineCtrl.method('circle').setVelocity(stepVelocity).getFullStep();
    end
    
    trajectory = r.transformSpline(trajectory);
    
    
    % Weight shift to base foot
    torso_delta = [0 weightShift 0];
    
    % Get trajectory of torso based on the weight shift. WeightShiftRatio
    % is zero --> torso on right foot, WeightShiftRatio is 1 --> torso on
    % left foot
    if(r.base == 1)
        weightShiftRatio = linspace(0.3,0.7,length(trajectory));
        % torso_delta(2) = abs(torso_delta(2));
    else
        weightShiftRatio = linspace(0.7,0.3,length(trajectory));
        % torso_delta(2) = -abs(torso_delta(2));
    end
    
    if(~stepType)
        torsoTrajectory = splineCtrl.getHalfWeightShift(torso_delta);
    else
        torsoTrajectory = splineCtrl.getFullWeightShift(torso_delta);
    end

    timeCurve = splineCtrl.getCustomEaseTimeCurve(0,1);
    
    i = i+1;
end
r.torso_z = torsoHeight;

r.point = [splineCtrl.easeTrajectory(trajectory(1,:),i,timeCurve)... 
    splineCtrl.easeTrajectory(trajectory(2,:),i,timeCurve)...
    splineCtrl.easeTrajectory(trajectory(3,:),i,timeCurve)];

r.step(0.5);

r.inverseKinematics();

q = r.q;

% Set final values as initial values for the next iteration
r.refresh();

% Reset iterator after we're done with the trajectory, otherwise we
% increment the counter and continue iterating as simulink continues
% sampling
if( i < (length(trajectory)))
    i = i+1;
else
    hold = 1;
end

end

== matlab function MARCH_demo/Controllers/Home/MATLAB Function ==
  data: q_i input size=[1 6]; done output double; samples input; wait input; q output; reset input
function [done,q] = fcn(q_i, samples,wait, reset)
%#codegen

persistent r splineCtrl i q_t j resetPersistent n q_f;

%% Initialize all variables
if(isempty(splineCtrl))
    splineCtrl = splineController();
    r = robotics();
end

if(isempty(q_t))
    q_t = [0 0 0 0 0 0];
    q_f = [0 0 0 0 0 0];
end

if(isempty(resetPersistent))
   resetPersistent = 0; 
end

if(isempty(i))
    i = 0;
    j = 0;
    n = 0;
end

%% Wait for motors
done = 0;
if( j <= wait)
   j=j+1;
   q = q_i;
   return;    
end


%% Logic
done = 0;

if(reset)
   i = 0;
end

if(n == 0)
    r.base = 1;
    r.inverseKinematics();
    q_f = r.q;
    n = 1;
end

% Run startup procedure
if(n == 1 && i == 0)
    splineCtrl.samples = samples;
    q_t = splineCtrl.getJointTrajectory(q_i,q_f);
    
    i = i+1;
end

q = q_t(i,:);

if(i < length(q_t))
    i = i+1;
else
    done = 1;
end

end

== matlab function MARCH_demo/State Machine/Create peak3/Greater than 0 ==
  data: peak input; signal output
function signal  = fcn(peak)


if peak >= 0
    signal = peak;
else
    signal = 0;
    
    
end

== matlab function MARCH_demo/EtherCAT Joint Setpoints/exoskeleton/MATLAB Function ==
  data: jointAngle input; encVal output; par parameter
function encVal = convertToEncoderValues(jointAngle, par)
encVal = zeros(6,1);

for i = 1:6
    encVal(i) = rad2enc(jointAngle(i), i, par);
end

== stateflow chart MARCH_demo/State Machine/State Machine ==
  state ZeroTorque
    en: controllerIndex = 1;
    en: action = 0;
    en: base = 0;
    en: stepType = 0;
    en: state = 1;
    continuous = 0;
    actionLocal = 0;
  state Homing
    en: controllerIndex = 2;
    en: action = 0;
    en: base = 0;
    en: stepType = 0;
    en: state = 2;
    continuous = 0;
  state ResetHome
    en: controllerIndex = 2;
    en: action = 1;
    en: base = 0;
    en: stepType = 0;
    en: state = 2;
  state HoldHome
    en: controllerIndex = 2;
    en: action = 0;
    en: base = 0;
    en: stepType = 0;
    en: state = 2;
    continuous = 0;
    baseLocal = 3;
  state DiscreteGait
    en: controllerIndex = 5;
    % We keep toggling the base with 4-baseLocal
    state standbyModeDiscr
      en: action = actionLocal;
      en: base = baseLocal;
      en: stepType = 0;
      en: state = 61;
      % Exoskeleton stands still in current position
    state startHalfStepCont
      en: action = 1;
      en: base = 4-baseLocal;
      en: stepType = 0;
      en: state = 6;
      baseLocal = base;
      continuous = 1;
    state startHalfStepDiscr
      en: action = 1;
      en: base = 4-baseLocal;
      en: stepType = 0;
      en: state = 6;
      baseLocal = base
    state leftFullStepDiscr
      en: action = action+1;
      en: base =  4-baseLocal;
      en: stepType = 1;
      en: state = 6;
      baseLocal = base;
      actionLocal = action;
    state rightFullStepDiscr
      en: action = action+1;
      en: base = 4-baseLocal;
      en: stepType = 1;
      en: state = 6;
      baseLocal = base;
      actionLocal = action;
    startHalfStepCont -> standbyModeDiscr [order 2] : [rightSafety ~=1 && done == 1]
    startHalfStepDiscr -> standbyModeDiscr [order 2] : [rightSafety ~=1 && done == 1]
    standbyModeDiscr -> rightFullStepDiscr [order 3] : [rightScrollMode == 4 && rightTrigger == 1 && rightSafety == 1]
    rightFullStepDiscr -> standbyModeDiscr [order 1] : [rightSafety ~=1 && done == 1]
    leftFullStepDiscr -> standbyModeDiscr [order 1] : [rightSafety ~=1 && done == 1]
    standbyModeDiscr -> leftFullStepDiscr [order 2] : [rightScrollMode == 3 && rightTrigger == 1 && rightSafety == 1]
    startHalfStepDiscr -> rightFullStepDiscr [order 1] : [done == 1 && rightTrigger == 1]
    startHalfStepCont -> rightFullStepDiscr [order 1] : [done == 1]
    rightFullStepDiscr -> leftFullStepDiscr [order 2] : [done == 1 && (rightTrigger ==  1 || continuous == 1)]
    leftFullStepDiscr -> rightFullStepDiscr [order 2] : [done == 1 && (rightTrigger ==  1 || continuous == 1)]
  (default) -> ZeroTorque
  ZeroTorque -> ResetHome : [rightScrollMode == 2]
  HoldHome -> ZeroTorque [order 3] : [rightScrollMode == 1]
  ResetHome -> Homing
  Homing -> HoldHome : [done == 1]
  standbyModeDiscr -> ResetHome [order 1] : [rightScrollMode == 2]
  HoldHome -> startHalfStepCont [order 2] : [rightScrollMode == 4 && rightTrigger == 1 && rightSafety == 1]
  HoldHome -> startHalfStepDiscr [order 1] : [rightScrollMode == 3 && rightTrigger == 1 && rightSafety == 1]
  data: rightTrigger input; rightSafety input; rightScrollMode input; rightScrollClick input; controllerIndex output; action output; base output; inpDevWorking local; done input; stepType output; state output; baseLocal local; actionLocal local; data local; continuous local
